simulink model "Segway"  (R2023b)
settings: Solver=FixedStepAuto  StartTime=0.0  StopTime=15  RelTol=1e-3
values from neighbouring files (symbols this model uses):
  C_input = 0.01    [parameters.m]
  dphi_0 = 0    [parameters.m]
  dx_0 = 0    [parameters.m]
  eom_params = struct('wheel_radius', wheel_radius,                  'body_mass', body_mass,                  'wheel_mass', wheel_mass,                  'semiaxis_wheels', semiaxis_wheels,                  'gravity', gravity,                  'center_of_mass', center_of_mass)    [parameters.m]
  freq_input = 1    [parameters.m]
  L_a1 = 1.6    [parameters.m]
  phi_0 = pi/2    (= 1.57079632679)    [parameters.m]
  S_a1 = 0.5    [parameters.m]
  std_dev_a1 = 1e-30    [parameters.m]
  std_dev_omega = 1e-10    [parameters.m]
  T_sensor_a1 = 0.033    [parameters.m]
  T_sensor_D = 0.025    [parameters.m]
  T_sensor_omega = 0.001    [parameters.m]
  x_0 = 0    [parameters.m]
settings Model: Creator=dario  LastModifiedBy=dario
settings OptimizationCC: ReuseModelBlockBuffer=off

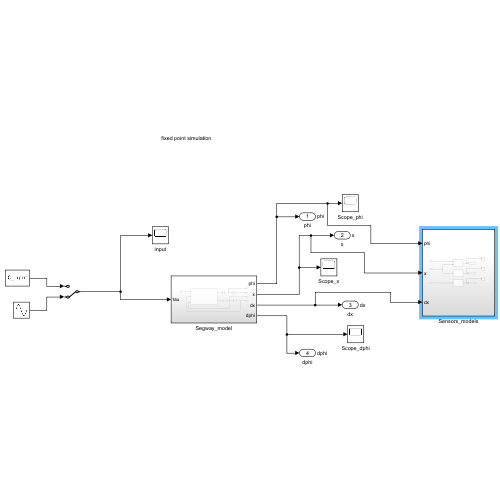
[thumbnail: Simulink's stored preview of the top-level diagram]
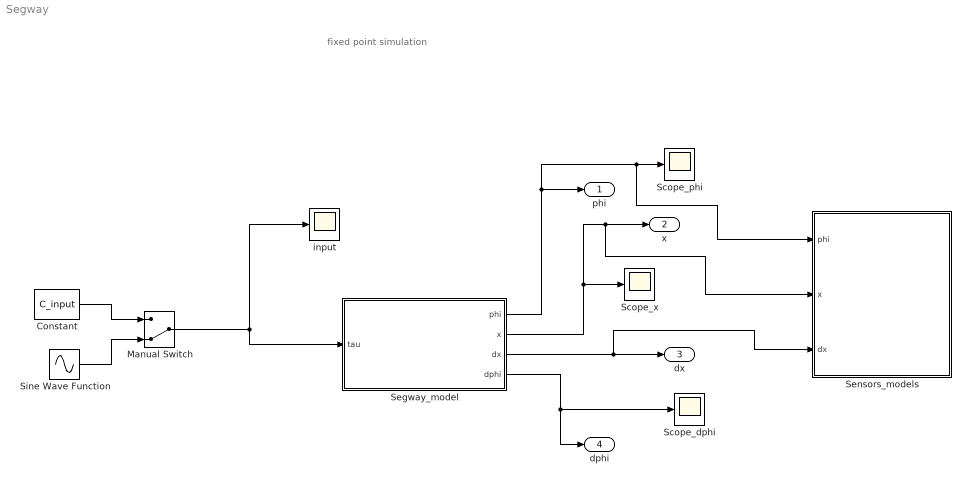
== system Segway ==
  note: fixed point simulation
  Constant : Constant  Value=C_input
  Manual Switch : ManualSwitch  CurrentSetting=0
  Scope_dphi : Scope
  Scope_phi : Scope
  Scope_x : Scope
  Segway_model : Subsystem
  Sensors_models : Subsystem
  Sine Wave Function : Sin  Amplitude=C_input  Frequency=freq_input  SampleTime=0
  input : Scope
  phi : Outport  SignalName=phi
  x : Outport  Port=2  SignalName=x
  dx : Outport  Port=3  SignalName=dx
  dphi : Outport  Port=4  SignalName=dphi
  wires:
  Manual Switch/1 -> input/1, Segway_model/1(tau)
  Segway_model/1(phi) -> Scope_phi/1, Sensors_models/1(phi), phi/1
  Segway_model/2(x) -> Sensors_models/2(x), x/1, Scope_x/1
  Segway_model/3(dx) -> Sensors_models/3(dx), dx/1
  Segway_model/4(dphi) -> Scope_dphi/1, dphi/1
  Sine Wave Function/1 -> Manual Switch/2
  Constant/1 -> Manual Switch/1

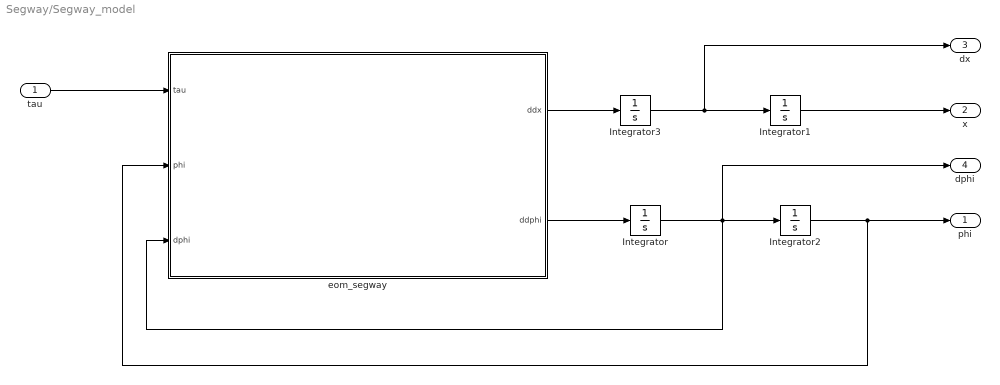
== system Segway/Segway_model ==
  tau : Inport
  Integrator : Integrator  InitialCondition=dphi_0
  Integrator1 : Integrator  InitialCondition=x_0
  Integrator2 : Integrator  InitialCondition=phi_0
  Integrator3 : Integrator  InitialCondition=dx_0
  eom_segway : MATLAB Function  TreatAsAtomicUnit=on
  phi : Outport
  x : Outport  Port=2
  dx : Outport  Port=3
  dphi : Outport  Port=4
  wires:
  tau/1 -> eom_segway/1(tau)
  Integrator1/1 -> x/1
  eom_segway/1(ddx) -> Integrator3/1
  Integrator2/1 -> phi/1, eom_segway/2(phi)
  Integrator/1 -> eom_segway/3(dphi), dphi/1, Integrator2/1
  Integrator3/1 -> dx/1, Integrator1/1
  eom_segway/2(ddphi) -> Integrator/1

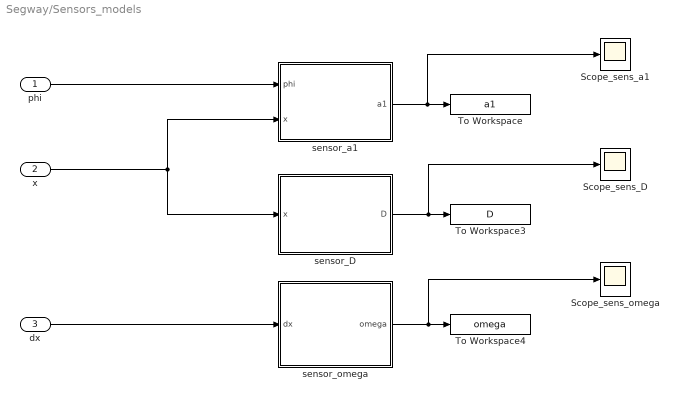
== system Segway/Sensors_models ==
  phi : Inport
  x : Inport  Port=2
  dx : Inport  Port=3
  Scope_sens_D : Scope
  Scope_sens_a1 : Scope
  Scope_sens_omega : Scope
  To Workspace : ToWorkspace  VariableName=a1  SaveFormat=Structure With Time  SampleTime=-1
  To Workspace3 : ToWorkspace  VariableName=D  SaveFormat=Structure With Time  SampleTime=-1
  To Workspace4 : ToWorkspace  VariableName=omega  SaveFormat=Structure With Time  SampleTime=-1
  sensor_D : MATLAB Function  TreatAsAtomicUnit=on  SystemSampleTime=T_sensor_D
  sensor_a1 : MATLAB Function  TreatAsAtomicUnit=on  SystemSampleTime=T_sensor_a1
  sensor_omega : MATLAB Function  TreatAsAtomicUnit=on  SystemSampleTime=T_sensor_omega
  wires:
  phi/1 -> sensor_a1/1(phi)
  sensor_omega/1(omega) -> Scope_sens_omega/1, To Workspace4/1
  x/1 -> sensor_a1/2(x), sensor_D/1(x)
  dx/1 -> sensor_omega/1(dx)
  sensor_a1/1(a1) -> Scope_sens_a1/1, To Workspace/1
  sensor_D/1(D) -> Scope_sens_D/1, To Workspace3/1

== matlab function Segway/Segway_model/eom_segway ==
  data: ddx output size=1; tau input; phi input; dphi input; ddphi output; eom_params parameter
% function that describes the EoM

function [ddx, ddphi] = eom_segway(tau, phi, dphi, eom_params)

% rename the parameters inside the struct
r = eom_params.wheel_radius;
mb = eom_params.body_mass;
mw = eom_params.wheel_mass;
g = eom_params.gravity;
L = eom_params.center_of_mass;
% a = eom_params.semiaxis_wheels; not used

% Operations in order to get the EoM
M_ddx = 2*(3/2*mw + 1/2*mb);
M_ddp = 2*(1/2*mw*r^2 + 2/3*mb*L^2);
M_ddxp = -mw*r + mb*L*cos(phi);
C_dx = -mb*L*sin(phi)*dphi^2;
g_p = -mb*g*L*sin(phi);

M = [M_ddx M_ddxp; M_ddxp M_ddp];
C = [C_dx 0]';
G = [0 g_p]';
C_tau = [2/r -2]';

q = M\(-C -G + C_tau*tau);

ddx = q(1);
ddphi = q(2);

== matlab function Segway/Sensors_models/sensor_D ==
  data: x input; D output; std_dev_D parameter
function D = sensor_D(x, std_dev_D)
% function to calculate the distance D
D = x + std_dev_D*randn(1,1);

== matlab function Segway/Sensors_models/sensor_omega ==
  data: dx input; omega output; std_dev_omega parameter; eom_params parameter
function omega = sensor_omega(dx, std_dev_omega, eom_params)
% function that calculates the angular velocity of the wheels
omega = 1/eom_params.wheel_radius * dx + std_dev_omega*randn(1,1);

== matlab function Segway/Sensors_models/sensor_a1 ==
  data: phi input; x input; a1 output; eom_params parameter; L_a1 parameter; S_a1 parameter; std_dev_a1 parameter
function a1 = sensor_a1(phi, x, eom_params, L_a1, S_a1, std_dev_a1)
% Function to calculate the angle a1
a1 = atan2(x - S_a1 + eom_params.center_of_mass*sin(phi),...
      L_a1 - eom_params.center_of_mass*cos(phi) - eom_params.wheel_radius) + std_dev_a1*randn(1,1);
